simulink model "SingleTrack"  (Simulink 10.3)
settings: Solver=ode45  StartTime=0.0  StopTime=inf  FixedStep=0.001  RelTol=1e-3
PreLoadFcn:
  | SingleTrack_params
undefined symbols (not defined in the file): Car_Bdy1_mass, Car_Steering_i, Car_Whl_Radius, Car_WhlBaseF, Car_WhlBaseR, mEngineMax, PT_DL_iDiff, PT_GearBox_iForwardGears
libraries: CarMaker4SL x9
(part 3 of 4)

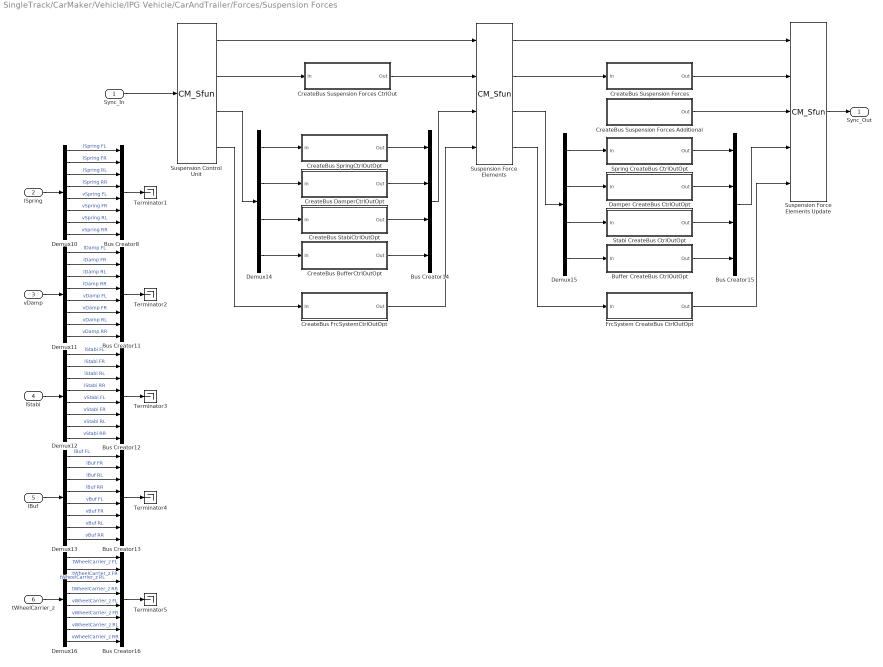
== system SingleTrack/CarMaker/Vehicle/IPG Vehicle/CarAndTrailer/Forces/Suspension Forces ==
  Sync_In : Inport
  lSpring : Inport  Port=2
  vDamp : Inport  Port=3
  lStabi : Inport  Port=4
  lBuf : Inport  Port=5
  tWheelCarrier_z : Inport  Port=6
  Buffer CreateBus CtrlOutOpt : Subsystem
  Bus Creator{8,11..13,16} (5 alike) : BusCreator  Inputs=8
  Bus Creator14 : BusCreator  Inputs=4
  Bus Creator15 : BusCreator  Inputs=4
  CreateBus BufferCtrlOutOpt : Subsystem
  CreateBus DamperCtrlOutOpt : Subsystem
  CreateBus FrcSystemCtrlOutOpt : Subsystem
  CreateBus SpringCtrlOutOpt : Subsystem
  CreateBus StabiCtrlOutOpt : Subsystem
  CreateBus Suspension Forces : Subsystem
  CreateBus Suspension Forces Additional : Subsystem
  CreateBus Suspension Forces CtrlOut : Subsystem
  Damper CreateBus CtrlOutOpt : Subsystem
  Demux{10..13,16} (5 alike) : Demux  Outputs=8
      settings: DisplayOption=none
  Demux14 : Demux
      settings: DisplayOption=none
  Demux15 : Demux
      settings: DisplayOption=none
  FrcSystem CreateBus CtrlOutOpt : Subsystem
  Spring CreateBus CtrlOutOpt : Subsystem
  Stabi CreateBus CtrlOutOpt : Subsystem
  Suspension Control Unit : S-Function  FunctionName=CM_Sfun  Parameters='ForcesSuspControl'  SFunctionDeploymentMode=off  EnableBusSupport=off
  Suspension Force Elements : S-Function  FunctionName=CM_Sfun  Parameters='ForcesSusp'  SFunctionDeploymentMode=off  EnableBusSupport=off
  Suspension Force Elements Update : S-Function  FunctionName=CM_Sfun  Parameters='ForcesSuspUpd'  SFunctionDeploymentMode=off  EnableBusSupport=off
  Terminator{1..5} (5 alike) : Terminator
  Sync_Out : Outport  VectorParamsAs1DForOutWhenUnconnected=off
  wires:
  Sync_In/1 -> Suspension Control Unit/1
  Suspension Control Unit/1 -> Suspension Force Elements/1
  Suspension Force Elements/1 -> Suspension Force Elements Update/1
  Suspension Force Elements Update/1 -> Sync_Out/1
  Demux13/4 -> Bus Creator13/4  "lBuf RR"
  Demux11/2 -> Bus Creator11/2  "lDamp FR"
  Demux13/8 -> Bus Creator13/8  "vBuf RR"
  Demux10/3 -> Bus Creator8/3  "lSpring RL"
  Demux10/1 -> Bus Creator8/1  "lSpring FL"
  vDamp/1 -> Demux11/1
  Demux13/2 -> Bus Creator13/2  "lBuf FR"
  Demux10/5 -> Bus Creator8/5  "vSpring FL"
  Bus Creator12/1 -> Terminator3/1
  Demux12/7 -> Bus Creator12/7  "vStabi RL"
  Demux10/4 -> Bus Creator8/4  "lSpring RR"
  Demux12/2 -> Bus Creator12/2  "lStabi FR"
  Demux11/5 -> Bus Creator11/5  "vDamp FL"
  Demux10/8 -> Bus Creator8/8  "vSpring RR"
  Demux12/1 -> Bus Creator12/1  "lStabi FL"
  Demux12/3 -> Bus Creator12/3  "lStabi RL"
  Demux11/6 -> Bus Creator11/6  "vDamp FR"
  lSpring/1 -> Demux10/1
  lBuf/1 -> Demux13/1
  Demux12/4 -> Bus Creator12/4  "lStabi RR"
  Bus Creator13/1 -> Terminator4/1
  Demux13/7 -> Bus Creator13/7  "vBuf RL"
  Demux12/8 -> Bus Creator12/8  "vStabi RR"
  Demux10/7 -> Bus Creator8/7  "vSpring RL"
  Demux11/8 -> Bus Creator11/8  "vDamp RR"
  Demux12/6 -> Bus Creator12/6  "vStabi FR"
  Demux11/1 -> Bus Creator11/1  "lDamp FL"
  Demux11/7 -> Bus Creator11/7  "vDamp RL"
  lStabi/1 -> Demux12/1
  Demux12/5 -> Bus Creator12/5  "vStabi FL"
  Bus Creator8/1 -> Terminator1/1
  Bus Creator11/1 -> Terminator2/1
  Demux13/1 -> Bus Creator13/1  "lBuf FL"
  Demux13/6 -> Bus Creator13/6  "vBuf FR"
  Demux11/4 -> Bus Creator11/4  "lDamp RR"
  Demux13/5 -> Bus Creator13/5  "vBuf FL"
  Demux10/6 -> Bus Creator8/6  "vSpring FR"
  Demux11/3 -> Bus Creator11/3  "lDamp RL"
  Demux10/2 -> Bus Creator8/2  "lSpring FR"
  Demux13/3 -> Bus Creator13/3  "lBuf RL"
  Suspension Force Elements/4 -> FrcSystem CreateBus CtrlOutOpt/1(In)
  FrcSystem CreateBus CtrlOutOpt/1(Out) -> Suspension Force Elements Update/5
  CreateBus SpringCtrlOutOpt/1(Out) -> Bus Creator14/1
  Demux14/1 -> CreateBus SpringCtrlOutOpt/1(In)
  Demux14/2 -> CreateBus DamperCtrlOutOpt/1(In)
  CreateBus DamperCtrlOutOpt/1(Out) -> Bus Creator14/2
  Demux14/3 -> CreateBus StabiCtrlOutOpt/1(In)
  CreateBus StabiCtrlOutOpt/1(Out) -> Bus Creator14/3
  CreateBus BufferCtrlOutOpt/1(Out) -> Bus Creator14/4
  Demux14/4 -> CreateBus BufferCtrlOutOpt/1(In)
  Demux15/4 -> Buffer CreateBus CtrlOutOpt/1(In)
  Buffer CreateBus CtrlOutOpt/1(Out) -> Bus Creator15/4
  Demux15/3 -> Stabi CreateBus CtrlOutOpt/1(In)
  Stabi CreateBus CtrlOutOpt/1(Out) -> Bus Creator15/3
  Demux15/2 -> Damper CreateBus CtrlOutOpt/1(In)
  Damper CreateBus CtrlOutOpt/1(Out) -> Bus Creator15/2
  Demux15/1 -> Spring CreateBus CtrlOutOpt/1(In)
  Spring CreateBus CtrlOutOpt/1(Out) -> Bus Creator15/1
  Suspension Force Elements/3 -> Demux15/1
  Bus Creator15/1 -> Suspension Force Elements Update/4
  Demux16/1 -> Bus Creator16/1  "tWheelCarrier_z FL"
  Demux16/6 -> Bus Creator16/6  "vWheelCarrier_z FR"
  Bus Creator16/1 -> Terminator5/1
  Demux16/2 -> Bus Creator16/2  "tWheelCarrier_z FR"
  Demux16/4 -> Bus Creator16/4  "tWheelCarrier_z RR"
  Demux16/8 -> Bus Creator16/8  "vWheelCarrier_z RR"
  Demux16/7 -> Bus Creator16/7  "vWheelCarrier_z RL"
  Demux16/3 -> Bus Creator16/3  "tWheelCarrier_z RL"
  Demux16/5 -> Bus Creator16/5  "vWheelCarrier_z FL"
  tWheelCarrier_z/1 -> Demux16/1
  CreateBus Suspension Forces Additional/1(Out) -> Suspension Force Elements Update/3
  Suspension Force Elements/2 -> CreateBus Suspension Forces/1(In)
  CreateBus Suspension Forces/1(Out) -> Suspension Force Elements Update/2
  Suspension Control Unit/2 -> CreateBus Suspension Forces CtrlOut/1(In)
  Suspension Control Unit/3 -> Demux14/1
  Suspension Control Unit/4 -> CreateBus FrcSystemCtrlOutOpt/1(In)
  CreateBus FrcSystemCtrlOutOpt/1(Out) -> Suspension Force Elements/4
  Bus Creator14/1 -> Suspension Force Elements/3
  CreateBus Suspension Forces CtrlOut/1(Out) -> Suspension Force Elements/2

== system SingleTrack/CarMaker/Vehicle/IPG Vehicle/CarAndTrailer/Forces/Tires ==
  note: The TireXX_Out signals will only be used if FileIdent is "CarMaker-Tire-CM4SL" in the tire parameter file!
      | An example parameter file can be found in Data/Tire/DT_CM4SL_UserTire.
  Sync_In : Inport
  TireFL_In : Inport  Port=2
  TireFR_In : Inport  Port=3
  TireRL_In : Inport  Port=4
  TireRR_In : Inport  Port=5
  Bus Creator{1..4} (4 alike) : BusCreator  Inputs=11
  Demux{1..3,8} (4 alike) : Demux  Outputs=7
      settings: DisplayOption=none
  TireFL : Subsystem
  TireFR : Subsystem
  TireRL : Subsystem
  TireRR : Subsystem
  TireFL_Out : Outport  VectorParamsAs1DForOutWhenUnconnected=off
  TireFR_Out : Outport  Port=2  VectorParamsAs1DForOutWhenUnconnected=off
  TireRL_Out : Outport  Port=3  VectorParamsAs1DForOutWhenUnconnected=off
  TireRR_Out : Outport  Port=4  VectorParamsAs1DForOutWhenUnconnected=off
  wires:
  Sync_In/1 -> TireRR/1(Sync_In), TireRL/1(Sync_In), TireFR/1(Sync_In), TireFL/1(Sync_In)
  Bus Creator4/1 -> TireRR_Out/1
  Bus Creator2/1 -> TireRL_Out/1
  Bus Creator1/1 -> TireFR_Out/1
  Demux3/5 -> TireRR/6(Rim_turnv)  "Tire_In Rim_turnv"
  Demux3/4 -> TireRR/5(Rim_rotv)  "Tire_In Rim_rotv"
  Demux3/1 -> TireRR/2(Load)  "Tire_In Load"
  Demux3/7 -> TireRR/8(muRoad)  "Tire_In mu"
  Demux3/6 -> TireRR/7(InclinAngle)  "Tire_In Camber"
  Demux3/2 -> TireRR/3(vxtrans)  "Tire_In vxtrans"
  Demux3/3 -> TireRR/4(vytrans)  "Tire_In vytrans"
  TireRR/11(AlignTrq) -> Bus Creator4/11  "Tire_Out AlignTrq"
  TireRR/10(RollResist) -> Bus Creator4/10  "Tire_Out RollResist"
  TireRR/9(OverturnTrq) -> Bus Creator4/9  "Tire_Out OverturnTrq"
  TireRR/8(LoadFrc) -> Bus Creator4/8  "Tire_Out LoadFrc"
  TireRR/7(SideFrc) -> Bus Creator4/7  "Tire_Out SideFrc"
  TireRR/6(LongFrc) -> Bus Creator4/6  "Tire_Out LongFrc"
  TireRR/5(vBelt) -> Bus Creator4/5  "Tire_Out vBelt"
  TireRR/4(rBelt_eff) -> Bus Creator4/4  "Tire_Out rBelt_eff"
  TireRR/3(TurnSlp) -> Bus Creator4/3  "Tire_Out TurnSlp"
  TireRR/1(Slp) -> Bus Creator4/1  "Tire_Out Slp"
  TireRR/2(Alpha) -> Bus Creator4/2  "Tire_Out Alpha"
  Demux2/5 -> TireRL/6(Rim_turnv)  "Tire_In Rim_turnv"
  Demux2/4 -> TireRL/5(Rim_rotv)  "Tire_In Rim_rotv"
  Demux2/1 -> TireRL/2(Load)  "Tire_In Load"
  Demux2/7 -> TireRL/8(muRoad)  "Tire_In mu"
  Demux2/6 -> TireRL/7(InclinAngle)  "Tire_In Camber"
  Demux2/2 -> TireRL/3(vxtrans)  "Tire_In vxtrans"
  Demux2/3 -> TireRL/4(vytrans)  "Tire_In vytrans"
  TireRL/11(AlignTrq) -> Bus Creator2/11  "Tire_Out AlignTrq"
  TireRL/10(RollResist) -> Bus Creator2/10  "Tire_Out RollResist"
  TireRL/9(OverturnTrq) -> Bus Creator2/9  "Tire_Out OverturnTrq"
  TireRL/8(LoadFrc) -> Bus Creator2/8  "Tire_Out LoadFrc"
  TireRL/7(SideFrc) -> Bus Creator2/7  "Tire_Out SideFrc"
  TireRL/6(LongFrc) -> Bus Creator2/6  "Tire_Out LongFrc"
  TireRL/5(vBelt) -> Bus Creator2/5  "Tire_Out vBelt"
  TireRL/4(rBelt_eff) -> Bus Creator2/4  "Tire_Out rBelt_eff"
  TireRL/3(TurnSlp) -> Bus Creator2/3  "Tire_Out TurnSlp"
  TireRL/1(Slp) -> Bus Creator2/1  "Tire_Out Slp"
  TireRL/2(Alpha) -> Bus Creator2/2  "Tire_Out Alpha"
  Demux1/5 -> TireFR/6(Rim_turnv)  "Tire_In Rim_turnv"
  Demux1/4 -> TireFR/5(Rim_rotv)  "Tire_In Rim_rotv"
  Demux1/1 -> TireFR/2(Load)  "Tire_In Load"
  Demux1/7 -> TireFR/8(muRoad)  "Tire_In mu"
  Demux1/6 -> TireFR/7(InclinAngle)  "Tire_In Camber"
  Demux1/2 -> TireFR/3(vxtrans)  "Tire_In vxtrans"
  Demux1/3 -> TireFR/4(vytrans)  "Tire_In vytrans"
  TireFR/11(AlignTrq) -> Bus Creator1/11  "Tire_Out AlignTrq"
  TireFR/10(RollResist) -> Bus Creator1/10  "Tire_Out RollResist"
  TireFR/9(OverturnTrq) -> Bus Creator1/9  "Tire_Out OverturnTrq"
  TireFR/8(LoadFrc) -> Bus Creator1/8  "Tire_Out LoadFrc"
  TireFR/7(SideFrc) -> Bus Creator1/7  "Tire_Out SideFrc"
  TireFR/6(LongFrc) -> Bus Creator1/6  "Tire_Out LongFrc"
  TireFR/5(vBelt) -> Bus Creator1/5  "Tire_Out vBelt"
  TireFR/4(rBelt_eff) -> Bus Creator1/4  "Tire_Out rBelt_eff"
  TireFR/3(TurnSlp) -> Bus Creator1/3  "Tire_Out TurnSlp"
  TireFR/1(Slp) -> Bus Creator1/1  "Tire_Out Slp"
  TireFR/2(Alpha) -> Bus Creator1/2  "Tire_Out Alpha"
  Demux8/5 -> TireFL/6(Rim_turnv)  "Tire_In Rim_turnv"
  Demux8/4 -> TireFL/5(Rim_rotv)  "Tire_In Rim_rotv"
  TireFL_In/1 -> Demux8/1
  Demux8/1 -> TireFL/2(Load)  "Tire_In Load"
  Demux8/7 -> TireFL/8(muRoad)  "Tire_In mu"
  Demux8/6 -> TireFL/7(InclinAngle)  "Tire_In Camber"
  Demux8/2 -> TireFL/3(vxtrans)  "Tire_In vxtrans"
  Demux8/3 -> TireFL/4(vytrans)  "Tire_In vytrans"
  TireFL/11(AlignTrq) -> Bus Creator3/11  "Tire_Out AlignTrq"
  TireFL/10(RollResist) -> Bus Creator3/10  "Tire_Out RollResist"
  TireFL/9(OverturnTrq) -> Bus Creator3/9  "Tire_Out OverturnTrq"
  TireFL/8(LoadFrc) -> Bus Creator3/8  "Tire_Out LoadFrc"
  TireFL/7(SideFrc) -> Bus Creator3/7  "Tire_Out SideFrc"
  TireFL/6(LongFrc) -> Bus Creator3/6  "Tire_Out LongFrc"
  TireFL/5(vBelt) -> Bus Creator3/5  "Tire_Out vBelt"
  TireFL/4(rBelt_eff) -> Bus Creator3/4  "Tire_Out rBelt_eff"
  TireFL/3(TurnSlp) -> Bus Creator3/3  "Tire_Out TurnSlp"
  TireFL/1(Slp) -> Bus Creator3/1  "Tire_Out Slp"
  TireFL/2(Alpha) -> Bus Creator3/2  "Tire_Out Alpha"
  Bus Creator3/1 -> TireFL_Out/1
  TireFR_In/1 -> Demux1/1
  TireRL_In/1 -> Demux2/1
  TireRR_In/1 -> Demux3/1

== system SingleTrack/CarMaker/Vehicle/IPG Vehicle/CarAndTrailer/Forces/Vehicle Forces ==
  Sync_In : Inport
  Bus Creator1 : BusCreator  Inputs=12
  Bus Creator8 : BusCreator  Inputs=16
  BusCreator1 : BusCreator  Inputs=4
  BusCreator2 : BusCreator  Inputs=9
  Demux : Demux  Outputs=16
      settings: DisplayOption=none
  Demux1 : Demux  Outputs=12
      settings: DisplayOption=none
  Demux2 : Demux  Outputs=13
      settings: DisplayOption=none
  Forces : S-Function  FunctionName=CM_Sfun  Parameters='Forces'  SFunctionDeploymentMode=off  EnableBusSupport=off
  Terminator : Terminator
  Sync_Out : Outport  VectorParamsAs1DForOutWhenUnconnected=off
  Car.Virtual : Outport  Port=2  VectorParamsAs1DForOutWhenUnconnected=off
  Car.Aero : Outport  Port=3  VectorParamsAs1DForOutWhenUnconnected=off
  Car.Load : Outport  Port=4  VectorParamsAs1DForOutWhenUnconnected=off
  wires:
  BusCreator1/1 -> Terminator/1  "Aero IF (in)"
  Demux2/13 -> BusCreator2/9  "car Aero Trq_1 z"
  Demux2/12 -> BusCreator2/8  "car Aero Trq_1 y"
  Demux2/11 -> BusCreator2/7  "car Aero Trq_1 x"
  Demux2/10 -> BusCreator2/6  "car Aero Frc_1 z"
  Demux2/9 -> BusCreator2/5  "car Aero Frc_1 y"
  Demux2/8 -> BusCreator2/4  "car Aero Frc_1 x"
  Demux2/7 -> BusCreator2/3  "car Aero PoA_1 z"
  Demux2/6 -> BusCreator2/2  "car Aero PoA_1 y"
  Demux2/5 -> BusCreator2/1  "car Aero PoA_1 x"
  Demux2/4 -> BusCreator1/4  "car Aero tau_1"
  Demux2/3 -> BusCreator1/3  "car Aero ApproachVel_1 z"
  Demux2/2 -> BusCreator1/2  "car Aero ApproachVel_1 y"
  Demux2/1 -> BusCreator1/1  "car Aero ApproachVel_1 x"
  Demux/16 -> Bus Creator8/16  "Car Load_3 tz"
  Demux/15 -> Bus Creator8/15  "Car Load_3 ty"
  Demux/14 -> Bus Creator8/14  "Car Load_3 tx"
  Demux/13 -> Bus Creator8/13  "Car Load_3 mass"
  Demux1/12 -> Bus Creator1/12  "Car Virtual Trq_0 z"
  Demux1/11 -> Bus Creator1/11  "Car Virtual Trq_0 y"
  Demux1/10 -> Bus Creator1/10  "Car Virtual Trq_0 x"
  Demux1/9 -> Bus Creator1/9  "Car Virtual Trq_1 z"
  Demux1/8 -> Bus Creator1/8  "Car Virtual Trq_1 y"
  Demux1/7 -> Bus Creator1/7  "Car Virtual Trq_1 x"
  Demux1/6 -> Bus Creator1/6  "Car Virtual Frc_0 z"
  Demux1/5 -> Bus Creator1/5  "Car Virtual Frc_0 y"
  Demux1/4 -> Bus Creator1/4  "Car Virtual Frc_0 x"
  Sync_In/1 -> Forces/1
  Forces/1 -> Sync_Out/1
  BusCreator2/1 -> Car.Aero/1
  Demux1/1 -> Bus Creator1/1  "Car Virtual Frc_1 x"
  Demux1/2 -> Bus Creator1/2  "Car Virtual Frc_1 y"
  Demux1/3 -> Bus Creator1/3  "Car Virtual Frc_1 z"
  Forces/3 -> Demux2/1
  Forces/2 -> Demux1/1
  Bus Creator1/1 -> Car.Virtual/1
  Bus Creator8/1 -> Car.Load/1
  Demux/1 -> Bus Creator8/1  "Car Load_0 mass"
  Demux/2 -> Bus Creator8/2  "Car Load_0 tx"
  Demux/3 -> Bus Creator8/3  "Car Load_0 ty"
  Demux/4 -> Bus Creator8/4  "Car Load_0 tz"
  Demux/5 -> Bus Creator8/5  "Car Load_1 mass"
  Demux/6 -> Bus Creator8/6  "Car Load_1 tx"
  Demux/7 -> Bus Creator8/7  "Car Load_1 ty"
  Demux/8 -> Bus Creator8/8  "Car Load_1 tz"
  Demux/9 -> Bus Creator8/9  "Car Load_2 mass"
  Demux/10 -> Bus Creator8/10  "Car Load_2 tx"
  Demux/11 -> Bus Creator8/11  "Car Load_2 ty"
  Demux/12 -> Bus Creator8/12  "Car Load_2 tz"
  Forces/4 -> Demux/1

== system SingleTrack/CarMaker/Vehicle/IPG Vehicle/CarAndTrailer/Trailer/CreateBus Car.Hitch.FrcTrq ==
  In1 : Inport
  Bus Creator7 : BusCreator  Inputs=6
  Demux7 : Demux  Outputs=6
      settings: DisplayOption=none
  Out1 : Outport  VectorParamsAs1DForOutWhenUnconnected=off
  wires:
  In1/1 -> Demux7/1
  Bus Creator7/1 -> Out1/1
  Demux7/6 -> Bus Creator7/6  "Car Hitch Trq2Car z"
  Demux7/5 -> Bus Creator7/5  "Car Hitch Trq2Car y"
  Demux7/4 -> Bus Creator7/4  "Car Hitch Trq2Car x"
  Demux7/3 -> Bus Creator7/3  "Car Hitch Frc2Car z"
  Demux7/2 -> Bus Creator7/2  "Car Hitch Frc2Car y"
  Demux7/1 -> Bus Creator7/1  "Car Hitch Frc2Car x"

== system SingleTrack/CarMaker/Vehicle/IPG Vehicle/CarAndTrailer/Trailer/CreateBus Vhcl.Motion ==
  In1 : Inport
  BusCreator : BusCreator  Inputs=15
  Demux : Demux  Outputs=15
      settings: DisplayOption=none
  Out1 : Outport  VectorParamsAs1DForOutWhenUnconnected=off
  wires:
  Demux/15 -> BusCreator/15  "Vhcl YawAcc"
  Demux/14 -> BusCreator/14  "Vhcl YawVel"
  Demux/13 -> BusCreator/13  "Vhcl Yaw"
  Demux/12 -> BusCreator/12  "Vhcl PitchAcc"
  Demux/11 -> BusCreator/11  "Vhcl PitchVel"
  Demux/10 -> BusCreator/10  "Vhcl Pitch"
  Demux/9 -> BusCreator/9  "Vhcl RollAcc"
  Demux/8 -> BusCreator/8  "Vhcl RollVel"
  Demux/7 -> BusCreator/7  "Vhcl Roll"
  Demux/6 -> BusCreator/6  "Vhcl Hitch_Pos z"
  Demux/5 -> BusCreator/5  "Vhcl Hitch_Pos y"
  Demux/4 -> BusCreator/4  "Vhcl Hitch_Pos x"
  Demux/3 -> BusCreator/3  "Vhcl sRoad"
  Demux/2 -> BusCreator/2  "Vhcl Distance"
  Demux/1 -> BusCreator/1  "Vhcl v"
  In1/1 -> Demux/1
  BusCreator/1 -> Out1/1

== system SingleTrack/CarMaker/Vehicle/IPG Vehicle/CarAndTrailer/Trailer/CreateBus Vhcl.PoI ==
  In1 : Inport
  Bus Creator3 : BusCreator  Inputs=18
  Demux3 : Demux  Outputs=18
      settings: DisplayOption=none
  Out1 : Outport  VectorParamsAs1DForOutWhenUnconnected=off
  wires:
  Demux3/18 -> Bus Creator3/18  "Vhcl PoI_GCS Elev"
  Demux3/17 -> Bus Creator3/17  "Vhcl PoI_GCS Lat"
  Demux3/16 -> Bus Creator3/16  "Vhcl PoI_GCS Long"
  Demux3/15 -> Bus Creator3/15  "Vhcl PoI_Acc_1 z"
  Demux3/14 -> Bus Creator3/14  "Vhcl PoI_Acc_1 y"
  Demux3/13 -> Bus Creator3/13  "Vhcl PoI_Acc_1 x"
  Demux3/12 -> Bus Creator3/12  "Vhcl PoI_Vel_1 z"
  Demux3/11 -> Bus Creator3/11  "Vhcl PoI_Vel_1 y"
  Demux3/10 -> Bus Creator3/10  "Vhcl PoI_Vel_1 x"
  Demux3/9 -> Bus Creator3/9  "Vhcl PoI_Acc z"
  Demux3/8 -> Bus Creator3/8  "Vhcl PoI_Acc y"
  Demux3/7 -> Bus Creator3/7  "Vhcl PoI_Acc x"
  Demux3/6 -> Bus Creator3/6  "Vhcl PoI_Vel z"
  Demux3/5 -> Bus Creator3/5  "Vhcl PoI_Vel y"
  Demux3/4 -> Bus Creator3/4  "Vhcl PoI_Vel x"
  Demux3/3 -> Bus Creator3/3  "Vhcl PoI_Pos z"
  Demux3/2 -> Bus Creator3/2  "Vhcl PoI_Pos y"
  In1/1 -> Demux3/1
  Bus Creator3/1 -> Out1/1
  Demux3/1 -> Bus Creator3/1  "Vhcl PoI_Pos x"

== system SingleTrack/CarMaker/Vehicle/IPG Vehicle/CarAndTrailer/Trailer/CreateBus Vhcl.Steering ==
  In1 : Inport
  Bus Creator3 : BusCreator  Inputs=4
  Demux : Demux
      settings: DisplayOption=none
  Out1 : Outport  VectorParamsAs1DForOutWhenUnconnected=off
  wires:
  Bus Creator3/1 -> Out1/1
  Demux/1 -> Bus Creator3/1  "Vhcl Steering Ang"
  Demux/3 -> Bus Creator3/3  "Vhcl Steering AngAcc"
  Demux/2 -> Bus Creator3/2  "Vhcl Steering AngVel"
  Demux/4 -> Bus Creator3/4  "Vhcl Steering Trq"
  In1/1 -> Demux/1

== system SingleTrack/CarMaker/Vehicle/IPG Vehicle/CarAndTrailer/Trailer/CreateBus Vhcl.Wheel.FL ==
  In1 : Inport
  Bus Creator3 : BusCreator  Inputs=14
  Demux3 : Demux  Outputs=14
      settings: DisplayOption=none
  Out1 : Outport  VectorParamsAs1DForOutWhenUnconnected=off
  wires:
  Demux3/14 -> Bus Creator3/14  "Vhcl Wheel FL Trq_WhlBearing"
  Demux3/13 -> Bus Creator3/13  "Vhcl Wheel FL Trq_T2W"
  Demux3/12 -> Bus Creator3/12  "Vhcl Wheel FL SideSlip"
  Demux3/11 -> Bus Creator3/11  "Vhcl Wheel FL LongSlip"
  Demux3/10 -> Bus Creator3/10  "Vhcl Wheel FL vBelt"
  Demux3/9 -> Bus Creator3/9  "Vhcl Wheel FL Fz"
  Demux3/8 -> Bus Creator3/8  "Vhcl Wheel FL Fy"
  Demux3/7 -> Bus Creator3/7  "Vhcl Wheel FL Fx"
  Demux3/6 -> Bus Creator3/6  "Vhcl Wheel FL r_zxy z"
  Demux3/5 -> Bus Creator3/5  "Vhcl Wheel FL r_zxy y"
  Demux3/4 -> Bus Creator3/4  "Vhcl Wheel FL r_zxy x"
  Demux3/3 -> Bus Creator3/3  "Vhcl Wheel FL t z"
  Demux3/2 -> Bus Creator3/2  "Vhcl Wheel FL t y"
  In1/1 -> Demux3/1
  Bus Creator3/1 -> Out1/1
  Demux3/1 -> Bus Creator3/1  "Vhcl Wheel FL t x"

== system SingleTrack/CarMaker/Vehicle/IPG Vehicle/CarAndTrailer/Trailer/CreateBus Vhcl.Wheel.FR ==
  In1 : Inport
  Bus Creator3 : BusCreator  Inputs=14
  Demux3 : Demux  Outputs=14
      settings: DisplayOption=none
  Out1 : Outport  VectorParamsAs1DForOutWhenUnconnected=off
  wires:
  Demux3/14 -> Bus Creator3/14  "Vhcl Wheel FR Trq_WhlBearing"
  Demux3/13 -> Bus Creator3/13  "Vhcl Wheel FR Trq_T2W"
  Demux3/12 -> Bus Creator3/12  "Vhcl Wheel FR SideSlip"
  Demux3/11 -> Bus Creator3/11  "Vhcl Wheel FR LongSlip"
  Demux3/10 -> Bus Creator3/10  "Vhcl Wheel FR vBelt"
  Demux3/9 -> Bus Creator3/9  "Vhcl Wheel FR Fz"
  Demux3/8 -> Bus Creator3/8  "Vhcl Wheel FR Fy"
  Demux3/7 -> Bus Creator3/7  "Vhcl Wheel FR Fx"
  Demux3/6 -> Bus Creator3/6  "Vhcl Wheel FR r_zxy z"
  Demux3/5 -> Bus Creator3/5  "Vhcl Wheel FR r_zxy y"
  Demux3/4 -> Bus Creator3/4  "Vhcl Wheel FR r_zxy x"
  Demux3/3 -> Bus Creator3/3  "Vhcl Wheel FR t z"
  Demux3/2 -> Bus Creator3/2  "Vhcl Wheel FR t y"
  In1/1 -> Demux3/1
  Bus Creator3/1 -> Out1/1
  Demux3/1 -> Bus Creator3/1  "Vhcl Wheel FR t x"

== system SingleTrack/CarMaker/Vehicle/IPG Vehicle/CarAndTrailer/Trailer/CreateBus Vhcl.Wheel.RL ==
  In1 : Inport
  Bus Creator3 : BusCreator  Inputs=14
  Demux3 : Demux  Outputs=14
      settings: DisplayOption=none
  Out1 : Outport  VectorParamsAs1DForOutWhenUnconnected=off
  wires:
  Demux3/14 -> Bus Creator3/14  "Vhcl Wheel RL Trq_WhlBearing"
  Demux3/13 -> Bus Creator3/13  "Vhcl Wheel RL Trq_T2W"
  Demux3/12 -> Bus Creator3/12  "Vhcl Wheel RL SideSlip"
  Demux3/11 -> Bus Creator3/11  "Vhcl Wheel RL LongSlip"
  Demux3/10 -> Bus Creator3/10  "Vhcl Wheel RL vBelt"
  Demux3/9 -> Bus Creator3/9  "Vhcl Wheel RL Fz"
  Demux3/8 -> Bus Creator3/8  "Vhcl Wheel RL Fy"
  Demux3/7 -> Bus Creator3/7  "Vhcl Wheel RL Fx"
  Demux3/6 -> Bus Creator3/6  "Vhcl Wheel RL r_zxy z"
  Demux3/5 -> Bus Creator3/5  "Vhcl Wheel RL r_zxy y"
  Demux3/4 -> Bus Creator3/4  "Vhcl Wheel RL r_zxy x"
  Demux3/3 -> Bus Creator3/3  "Vhcl Wheel RL t z"
  Demux3/2 -> Bus Creator3/2  "Vhcl Wheel RL t y"
  In1/1 -> Demux3/1
  Bus Creator3/1 -> Out1/1
  Demux3/1 -> Bus Creator3/1  "Vhcl Wheel RL t x"

== system SingleTrack/CarMaker/Vehicle/IPG Vehicle/CarAndTrailer/Trailer/CreateBus Vhcl.Wheel.RR ==
  In1 : Inport
  Bus Creator3 : BusCreator  Inputs=14
  Demux3 : Demux  Outputs=14
      settings: DisplayOption=none
  Out1 : Outport  VectorParamsAs1DForOutWhenUnconnected=off
  wires:
  Demux3/14 -> Bus Creator3/14  "Vhcl Wheel RR Trq_WhlBearing"
  Demux3/13 -> Bus Creator3/13  "Vhcl Wheel RR Trq_T2W"
  Demux3/12 -> Bus Creator3/12  "Vhcl Wheel RR SideSlip"
  Demux3/11 -> Bus Creator3/11  "Vhcl Wheel RR LongSlip"
  Demux3/10 -> Bus Creator3/10  "Vhcl Wheel RR vBelt"
  Demux3/9 -> Bus Creator3/9  "Vhcl Wheel RR Fz"
  Demux3/8 -> Bus Creator3/8  "Vhcl Wheel RR Fy"
  Demux3/7 -> Bus Creator3/7  "Vhcl Wheel RR Fx"
  Demux3/6 -> Bus Creator3/6  "Vhcl Wheel RR r_zxy z"
  Demux3/5 -> Bus Creator3/5  "Vhcl Wheel RR r_zxy y"
  Demux3/4 -> Bus Creator3/4  "Vhcl Wheel RR r_zxy x"
  Demux3/3 -> Bus Creator3/3  "Vhcl Wheel RR t z"
  Demux3/2 -> Bus Creator3/2  "Vhcl Wheel RR t y"
  In1/1 -> Demux3/1
  Bus Creator3/1 -> Out1/1
  Demux3/1 -> Bus Creator3/1  "Vhcl Wheel RR t x"

== system SingleTrack/CarMaker/Vehicle/User Vehicle (CM4SL)/CarAndTrailer/CarAndTrailerUpd/CreateBus Brake.IF.In ==
  In : Inport
  BusCreator : BusCreator  Inputs=9
  Demux : Demux  Outputs=9
      settings: DisplayOption=none
  Out : Outport  VectorParamsAs1DForOutWhenUnconnected=off
  wires:
  Demux/9 -> BusCreator/9  "Brake IF Trq_Reg RR"
  Demux/8 -> BusCreator/8  "Brake IF Trq_Reg RL"
  Demux/7 -> BusCreator/7  "Brake IF Trq_Reg FR"
  Demux/6 -> BusCreator/6  "Brake IF Trq_Reg FL"
  Demux/5 -> BusCreator/5  "Brake IF Trq_Reg_max RR"
  Demux/4 -> BusCreator/4  "Brake IF Trq_Reg_max RL"
  Demux/3 -> BusCreator/3  "Brake IF Trq_Reg_max FR"
  Demux/2 -> BusCreator/2  "Brake IF Trq_Reg_max FL"
  Demux/1 -> BusCreator/1  "Brake IF T_env"
  BusCreator/1 -> Out/1
  In/1 -> Demux/1

== system SingleTrack/CarMaker/Vehicle/User Vehicle (CM4SL)/CarAndTrailer/CreateBus Vhcl.Fr1/BdyFrame2Vhcl.Fr1A ==
  note: Translate pseudo BdyFrame interface to Vhcl.Fr1
  t_0 : Inport
  v_0 : Inport  Port=2
  a_0 : Inport  Port=3
  omega_0 : Inport  Port=4
  alpha_0 : Inport  Port=5
  Tr2Fr0 : Inport  Port=6
  Bus Creator : BusCreator  Inputs=24
  Demux{,1..3,5} (5 alike) : Demux  Outputs=3
  Demux4 : Demux  Outputs=9
  Vhcl.Fr1 : Outport  VectorParamsAs1DForOutWhenUnconnected=off
  wires:
  t_0/1 -> Demux/1
  v_0/1 -> Demux1/1
  a_0/1 -> Demux2/1
  omega_0/1 -> Demux3/1
  alpha_0/1 -> Demux5/1
  Tr2Fr0/1 -> Demux4/1
  Demux4/9 -> Bus Creator/24  "Vhcl Fr1A_Tr2Fr0 22"
  Demux4/8 -> Bus Creator/23  "Vhcl Fr1A_Tr2Fr0 21"
  Demux4/7 -> Bus Creator/22  "Vhcl Fr1A_Tr2Fr0 20"
  Demux4/6 -> Bus Creator/21  "Vhcl Fr1A_Tr2Fr0 12"
  Demux4/5 -> Bus Creator/20  "Vhcl Fr1A_Tr2Fr0 11"
  Demux4/4 -> Bus Creator/19  "Vhcl Fr1A_Tr2Fr0 10"
  Demux4/3 -> Bus Creator/18  "Vhcl Fr1A_Tr2Fr0 02"
  Demux4/2 -> Bus Creator/17  "Vhcl Fr1A_Tr2Fr0 01"
  Demux4/1 -> Bus Creator/16  "Vhcl Fr1A_Tr2Fr0 00"
  Demux5/3 -> Bus Creator/15  "Vhcl Fr1A_alpha_0 z"
  Demux5/2 -> Bus Creator/14  "Vhcl Fr1A_alpha_0 y"
  Demux5/1 -> Bus Creator/13  "Vhcl Fr1A_alpha_0 x"
  Demux3/3 -> Bus Creator/12  "Vhcl Fr1A_omega_0 z"
  Demux3/2 -> Bus Creator/11  "Vhcl Fr1A_omega_0 y"
  Demux3/1 -> Bus Creator/10  "Vhcl Fr1A_omega_0 x"
  Demux2/3 -> Bus Creator/9  "Vhcl Fr1A_a_0 z"
  Demux2/2 -> Bus Creator/8  "Vhcl Fr1A_a_0 y"
  Demux2/1 -> Bus Creator/7  "Vhcl Fr1A_a_0 x"
  Demux1/3 -> Bus Creator/6  "Vhcl Fr1A_v_0 z"
  Demux1/2 -> Bus Creator/5  "Vhcl Fr1A_v_0 y"
  Demux1/1 -> Bus Creator/4  "Vhcl Fr1A_v_0 x"
  Demux/3 -> Bus Creator/3  "Vhcl Fr1A_t_0 z"
  Demux/2 -> Bus Creator/2  "Vhcl Fr1A_t_0 y"
  Demux/1 -> Bus Creator/1  "Vhcl Fr1 A_t_0 x"
  Bus Creator/1 -> Vhcl.Fr1/1

== system SingleTrack/CarMaker/Vehicle/User Vehicle (CM4SL)/CarAndTrailer/CreateBus Vhcl.Fr1/Tr2Fr0 ==
  Car : Inport
  Bus Creator : BusCreator  Inputs=9
  Subsystem_00 : Subsystem
  Subsystem_01 : Subsystem
  Subsystem_02 : Subsystem
  Subsystem_10 : Subsystem
  Subsystem_11 : Subsystem
  Subsystem_12 : Subsystem
  Subsystem_20 : Subsystem
  Subsystem_21 : Subsystem
  Subsystem_22 : Subsystem
  sincos : Subsystem
  Tr2Fr0 : Outport  VectorParamsAs1DForOutWhenUnconnected=off
  wires:
  Car/1 -> sincos/1(Car)
  sincos/1(sincos) -> Subsystem_10/1(sincos), Subsystem_11/1(sincos), Subsystem_20/1(sincos), Subsystem_21/1(sincos), Subsystem_22/1(sincos), Subsystem_12/1(sincos), Subsystem_00/1(sincos), Subsystem_01/1(sincos), Subsystem_02/1(sincos)
  Bus Creator/1 -> Tr2Fr0/1
  Subsystem_00/1(Tr2Fr1_00) -> Bus Creator/1  "Tr2Fr0_00"
  Subsystem_10/1(Tr2Fr1_10) -> Bus Creator/4  "Tr2Fr0_10"
  Subsystem_20/1(Tr2Fr1_20) -> Bus Creator/7  "Tr2Fr0_20"
  Subsystem_21/1(Tr2Fr1_21) -> Bus Creator/8  "Tr2Fr0_21"
  Subsystem_22/1(Tr2Fr1_22) -> Bus Creator/9  "Tr2Fr0_22"
  Subsystem_01/1(Tr2Fr1_01) -> Bus Creator/2  "Tr2Fr0_01"
  Subsystem_02/1(Tr2Fr1_02) -> Bus Creator/3  "Tr2Fr0_02"
  Subsystem_11/1(Tr2Fr1_11) -> Bus Creator/5  "Tr2Fr1_11"
  Subsystem_12/1(Tr2Fr1_12) -> Bus Creator/6  "Tr2Fr1_12"

== system SingleTrack/CarMaker/Vehicle/User Vehicle (CM4SL)/CarAndTrailer/CreateBus Vhcl.Fr1/a_0 ==
  Car : Inport
  Tr2Fr0 : Inport  Port=2
  Add : Sum
  Add1 : Sum
  Add2 : Sum
  Bus Selector1 : BusSelector  OutputSignals=Car_ax_1,Car_ay_1
  Bus Selector2 : BusSelector  OutputSignals=Tr2Fr0_00,Tr2Fr0_01,Tr2Fr0_10,Tr2Fr1_11,Tr2Fr0_20,Tr2Fr0_21
  Mux1 : Mux  Inputs=3
  Product{,1..5} (6 alike) : Product  RndMeth=Zero
  a_0 : Outport  VectorParamsAs1DForOutWhenUnconnected=off
  wires:
  Mux1/1 -> a_0/1
  Car/1 -> Bus Selector1/1
  Tr2Fr0/1 -> Bus Selector2/1
  Bus Selector1/2 -> Product/1, Product2/1, Product4/1  "<Car_ay_1>"
  Bus Selector1/1 -> Product1/1, Product3/1, Product5/1  "<Car_ax_1>"
  Product1/1 -> Add/1
  Product/1 -> Add/2
  Add/1 -> Mux1/1
  Product3/1 -> Add1/1
  Product2/1 -> Add1/2
  Bus Selector2/1 -> Product1/2  "<Tr2Fr0_00>"
  Bus Selector2/2 -> Product/2  "<Tr2Fr0_01>"
  Add1/1 -> Mux1/2
  Bus Selector2/3 -> Product3/2  "<Tr2Fr0_10>"
  Bus Selector2/4 -> Product2/2  "<Tr2Fr1_11>"
  Product5/1 -> Add2/1
  Product4/1 -> Add2/2
  Add2/1 -> Mux1/3
  Bus Selector2/6 -> Product4/2  "<Tr2Fr0_21>"
  Bus Selector2/5 -> Product5/2  "<Tr2Fr0_20>"

== system SingleTrack/CarMaker/Vehicle/User Vehicle (CM4SL)/CarAndTrailer/CreateBus Vhcl.Fr1/t_0 ==
  Car : Inport
  Bus Selector : BusSelector  OutputSignals=Car_x,Car_y,Road_Fr1_z
  Mux : Mux  Inputs=3
  t_0 : Outport  VectorParamsAs1DForOutWhenUnconnected=off
  wires:
  Bus Selector/1 -> Mux/1  "<Car_x>"
  Bus Selector/2 -> Mux/2  "<Car_y>"
  Bus Selector/3 -> Mux/3  "<Road_Fr1_z>"
  Car/1 -> Bus Selector/1
  Mux/1 -> t_0/1

== system SingleTrack/CarMaker/Vehicle/User Vehicle (CM4SL)/CarAndTrailer/CreateBus Vhcl.Fr1/v_0 ==
  Car : Inport
  Tr2Fr0 : Inport  Port=2
  Bus Selector1 : BusSelector  OutputSignals=Car_vx_1
  Bus Selector2 : BusSelector  OutputSignals=Tr2Fr0_00,Tr2Fr0_10,Tr2Fr0_20
  Mux1 : Mux  Inputs=3
  Product : Product  RndMeth=Zero
  Product1 : Product  RndMeth=Zero
  Product2 : Product  RndMeth=Zero
  v_0 : Outport  VectorParamsAs1DForOutWhenUnconnected=off
  wires:
  Car/1 -> Bus Selector1/1
  Mux1/1 -> v_0/1
  Tr2Fr0/1 -> Bus Selector2/1
  Bus Selector2/1 -> Product/2  "<Tr2Fr0_00>"
  Bus Selector2/2 -> Product1/2  "<Tr2Fr0_10>"
  Bus Selector2/3 -> Product2/2  "<Tr2Fr0_20>"
  Bus Selector1/1 -> Product/1, Product1/1, Product2/1  "<Car_vx_1>"
  Product/1 -> Mux1/1
  Product1/1 -> Mux1/2
  Product2/1 -> Mux1/3

== system SingleTrack/CarMaker/Vehicle/User Vehicle (CM4SL)/CarAndTrailer/PowerTrainUpd/Set OperationState ==
  note: Handles OperationState in Post-processing (SimCore.State >=9)
  If : If  IfExpression=u1 >= 9
  If Action Subsystem : Subsystem  TreatAsAtomicUnit=on
  If Action Subsystem1 : Subsystem  TreatAsAtomicUnit=on
  Merge : Merge
  Read CM Dict : CarMaker4SL/Read CM Dict  xname=SC.State  xsync=off  xstime=Continuous
  Read CM Dict1 : CarMaker4SL/Read CM Dict  xname=DM.OperationState_trg  xsync=off  xstime=Continuous
  OperationState : Outport  VectorParamsAs1DForOutWhenUnconnected=off
  wires:
  Merge/1 -> OperationState/1
  If/1 -> If Action Subsystem/Action
  If/2 -> If Action Subsystem1/Action
  If Action Subsystem/1(Out1) -> Merge/1
  If Action Subsystem1/1(Out1) -> Merge/2
  Read CM Dict/1 -> If/1
  Read CM Dict1/1 -> If Action Subsystem1/1(In1), If Action Subsystem/1(In1)

== system SingleTrack/CarMaker/Vehicle/User Vehicle (CM4SL)/CarAndTrailer/Query Road/IPGRoad5 ==
  rIn.st : Inport
  rIn.xyz : Inport  Port=2
  Bus Creator1 : BusCreator  Inputs=9
  Bus Creator2 : BusCreator  Inputs=22
  Demux1 : Demux  Outputs=9
  Demux3 : Demux  Outputs=22
  S-Function : S-Function  FunctionName=cm_road  Parameters=xname,xevalmode,xconsiderbumps,xusepath,xwithcurve,xabort  SFunctionDeploymentMode=off  EnableBusSupport=off
  rOutGeo : Outport  VectorParamsAs1DForOutWhenUnconnected=off
  rOutRoute : Outport  Port=2  VectorParamsAs1DForOutWhenUnconnected=off
  wires:
  Demux3/22 -> Bus Creator2/22  "fric"
  S-Function/2 -> Demux3/1
  S-Function/1 -> Demux1/1
  Bus Creator1/1 -> rOutGeo/1
  Demux1/9 -> Bus Creator1/9  "fric"
  Demux1/8 -> Bus Creator1/8  "onJunction"
  Demux1/7 -> Bus Creator1/7  "onRoad"
  Demux1/6 -> Bus Creator1/6  "nuv z"
  Demux1/5 -> Bus Creator1/5  "nuv y"
  Demux1/4 -> Bus Creator1/4  "nuv x"
  Demux1/3 -> Bus Creator1/3  "z"
  Demux1/2 -> Bus Creator1/2  "y"
  Demux1/1 -> Bus Creator1/1  "x"
  Demux3/21 -> Bus Creator2/21  "curveZ"
  Demux3/20 -> Bus Creator2/20  "slope"
  Demux3/19 -> Bus Creator2/19  "grade"
  Demux3/18 -> Bus Creator2/18  "onRoad"
  Demux3/17 -> Bus Creator2/17  "width right"
  Demux3/16 -> Bus Creator2/16  "width left"
  Demux3/15 -> Bus Creator2/15  "curveXY"
  Demux3/13 -> Bus Creator2/13  "s"
  Demux3/14 -> Bus Creator2/14  "t"
  Demux3/12 -> Bus Creator2/12  "tuv z"
  Demux3/11 -> Bus Creator2/11  "tuv y"
  Demux3/10 -> Bus Creator2/10  "tuv x"
  Demux3/9 -> Bus Creator2/9  "suv z"
  Demux3/8 -> Bus Creator2/8  "suv y"
  Demux3/7 -> Bus Creator2/7  "suv x"
  Demux3/6 -> Bus Creator2/6  "nuv z"
  Demux3/5 -> Bus Creator2/5  "nuv y"
  Demux3/4 -> Bus Creator2/4  "nuv x"
  Demux3/3 -> Bus Creator2/3  "z"
  Demux3/2 -> Bus Creator2/2  "y"
  Demux3/1 -> Bus Creator2/1  "x"
  Bus Creator2/1 -> rOutRoute/1
  rIn.xyz/1 -> S-Function/2
  rIn.st/1 -> S-Function/1

== system SingleTrack/CarMaker/Vehicle/User Vehicle (CM4SL)/CarAndTrailer/single-track mass point model/Car.v_1 ==
  ax : Inport
  Constant1 : Constant  Value=0.1
  PassIfSim : Subsystem
  Read CM Parameter : CarMaker4SL/Read CM Parameter  xfile=TestRun  xkey=DrivMan.Man.Start.Velocity  xnout=1  xdefaults=0  xmuxed=on  xstime=Continuous
  kmh2ms : Gain  Gain=1000/3600  OutDataTypeStr=Inherit: Inherit via back propagation  SaturateOnIntegerOverflow=on  ParamDataTypeStr=Inherit: Same as input
  vMin : MinMax  Function=max  Inputs=2  InputSameDT=on  SaturateOnIntegerOverflow=on
  v_dot * dt : Integrator  ExternalReset=level  InitialConditionSource=external  InitialCondition=22.222
  v_1 : Outport  VectorParamsAs1DForOutWhenUnconnected=off
  wires:
  Read CM Parameter/1 -> kmh2ms/1
  kmh2ms/1 -> vMin/2
  Constant1/1 -> vMin/1
  [TRStart] -> v_dot * dt/2
  vMin/1 -> v_dot * dt/3
  v_dot * dt/1 -> v_1/1
  ax/1 -> PassIfSim/1(In1)
  PassIfSim/1(Out1) -> v_dot * dt/1

== system SingleTrack/CarMaker/Vehicle/User Vehicle (CM4SL)/CarAndTrailer/single-track mass point model/PassIfSim ==
  note: Output original value only when simulating,
      | and zero during pre- or postprocessing.
  In1 : Inport
  "   " : Product  InputSameDT=on  SaturateOnIntegerOverflow=on  OutDataTypeStr=Inherit: Same as first input
  Data Type Conversion : DataTypeConversion
  Out1 : Outport  VectorParamsAs1DForOutWhenUnconnected=off
  wires:
  [TRSim] -> Data Type Conversion/1
  "   "/1 -> Out1/1
  Data Type Conversion/1 -> "   "/2
  In1/1 -> "   "/1

== system SingleTrack/CarMaker/Vehicle/User Vehicle (CM4SL)/CarAndTrailer/single-track mass point model/PassIfSim1 ==
  note: Output original value only when simulating,
      | and zero during pre- or postprocessing.
  In1 : Inport
  "   " : Product  InputSameDT=on  SaturateOnIntegerOverflow=on  OutDataTypeStr=Inherit: Same as first input
  Data Type Conversion : DataTypeConversion
  Out1 : Outport  VectorParamsAs1DForOutWhenUnconnected=off
  wires:
  [TRSim] -> Data Type Conversion/1
  "   "/1 -> Out1/1
  Data Type Conversion/1 -> "   "/2
  In1/1 -> "   "/1

== system SingleTrack/CarMaker/Vehicle/User Vehicle (CM4SL)/CarAndTrailer/single-track mass point model/PassIfSim2 ==
  note: Output original value only when simulating,
      | and zero during pre- or postprocessing.
  In1 : Inport
  "   " : Product  InputSameDT=on  SaturateOnIntegerOverflow=on  OutDataTypeStr=Inherit: Same as first input
  Data Type Conversion : DataTypeConversion
  Out1 : Outport  VectorParamsAs1DForOutWhenUnconnected=off
  wires:
  [TRSim] -> Data Type Conversion/1
  "   "/1 -> Out1/1
  Data Type Conversion/1 -> "   "/2
  In1/1 -> "   "/1

== system SingleTrack/CarMaker/Vehicle/User Vehicle (CM4SL)/CarAndTrailer/single-track mass point model/Vehicle Initial Cfg ==
  CreateBus Vhcl.Cfg : Subsystem
  VehicleControlUpd : S-Function  FunctionName=cm_initial  SFunctionDeploymentMode=off  EnableBusSupport=off
  Vhcl.Cfg : Outport  VectorParamsAs1DForOutWhenUnconnected=off
  wires:
  VehicleControlUpd/1 -> CreateBus Vhcl.Cfg/1(In1)
  CreateBus Vhcl.Cfg/1(Out1) -> Vhcl.Cfg/1

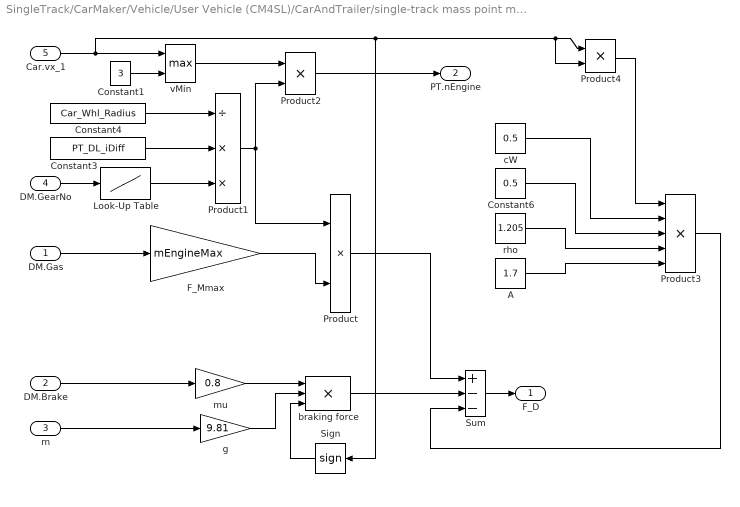
== system SingleTrack/CarMaker/Vehicle/User Vehicle (CM4SL)/CarAndTrailer/single-track mass point model/driving force ==
  DM.Gas : Inport
  DM.Brake : Inport  Port=2
  m : Inport  Port=3
  DM.GearNo : Inport  Port=4
  Car.vx_1 : Inport  Port=5
  A : Constant  Value=1.7
  Constant1 : Constant  Value=3
  Constant3 : Constant  Value=PT_DL_iDiff
  Constant4 : Constant  Value=Car_Whl_Radius
  Constant6 : Constant  Value=0.5
  "F_Mmax " : Gain  Gain=mEngineMax  SaturateOnIntegerOverflow=on  OutDataTypeStr=Inherit: Same as input  ParamDataTypeStr=Inherit: Same as input
  Look-Up Table : Lookup  InputValues=[0 1 2 3 4 5 6]  Table=PT_GearBox_iForwardGears  LookUpMeth=Interpolation-Use End Values  SaturateOnIntegerOverflow=on
  Product : Product  Inputs=**  InputSameDT=on  SaturateOnIntegerOverflow=on  OutDataTypeStr=Inherit: Same as first input
  Product1 : Product  Inputs=/**  InputSameDT=on  SaturateOnIntegerOverflow=on  OutDataTypeStr=Inherit: Same as first input
  Product2 : Product  InputSameDT=on  SaturateOnIntegerOverflow=on  OutDataTypeStr=Inherit: Same as first input
  Product3 : Product  Inputs=5  InputSameDT=on  SaturateOnIntegerOverflow=on  OutDataTypeStr=Inherit: Same as first input
  Product4 : Product  InputSameDT=on  SaturateOnIntegerOverflow=on  OutDataTypeStr=Inherit: Same as first input
  Sign : Signum  ZeroCross=off
  Sum : Sum  Inputs=+--  InputSameDT=on  SaturateOnIntegerOverflow=on  OutDataTypeStr=Inherit: Same as first input
  braking force : Product  Inputs=3  InputSameDT=on  SaturateOnIntegerOverflow=on  OutDataTypeStr=Inherit: Same as first input
  cW : Constant  Value=0.5
  g : Gain  Gain=9.81  SaturateOnIntegerOverflow=on  OutDataTypeStr=Inherit: Same as input  ParamDataTypeStr=Inherit: Same as input
  mu : Gain  Gain=0.8  SaturateOnIntegerOverflow=on  OutDataTypeStr=Inherit: Same as input  ParamDataTypeStr=Inherit: Same as input
  rho : Constant  Value=1.205
  vMin : MinMax  Function=max  Inputs=2  InputSameDT=on  SaturateOnIntegerOverflow=on
  F_D : Outport  VectorParamsAs1DForOutWhenUnconnected=off
  PT.nEngine : Outport  Port=2  VectorParamsAs1DForOutWhenUnconnected=off
  wires:
  Sign/1 -> braking force/3
  Product2/1 -> PT.nEngine/1
  vMin/1 -> Product2/1
  Constant1/1 -> vMin/2
  Car.vx_1/1 -> Sign/1, Product4/1, Product4/2, vMin/1
  DM.Brake/1 -> mu/1
  "F_Mmax "/1 -> Product/2
  Look-Up Table/1 -> Product1/3
  Product1/1 -> Product/1, Product2/2
  Constant4/1 -> Product1/1
  Constant3/1 -> Product1/2
  Product/1 -> Sum/1
  DM.GearNo/1 -> Look-Up Table/1
  Sum/1 -> F_D/1
  braking force/1 -> Sum/2
  g/1 -> braking force/2
  m/1 -> g/1
  mu/1 -> braking force/1
  DM.Gas/1 -> "F_Mmax "/1
  A/1 -> Product3/5
  rho/1 -> Product3/4
  Constant6/1 -> Product3/3
  cW/1 -> Product3/2
  Product4/1 -> Product3/1
  Product3/1 -> Sum/3

== system SingleTrack/CarMaker/Vehicle/User Vehicle (CM4SL)/CarAndTrailer/single-track mass point model/yaw ==
  Steer.Ang : Inport
  Car.v : Inport  Port=2
  Car.v_dot : Inport  Port=3
  Car.mass : Inport  Port=4
  1/ J : Gain  Gain=1/1322.5  SaturateOnIntegerOverflow=on  OutDataTypeStr=Inherit: Same as input  ParamDataTypeStr=Inherit: Same as input
  Bus Selector : BusSelector  OutputSignals=Vhcl Cfg Yaw
  Multiply : Product  Inputs=**  OutDataTypeStr=double
  Sum : Sum  Inputs=+-  InputSameDT=on  SaturateOnIntegerOverflow=on  OutDataTypeStr=Inherit: Same as first input
  Sum1 : Sum  InputSameDT=on  SaturateOnIntegerOverflow=on  OutDataTypeStr=Inherit: Same as first input
  Vehicle Initial Cfg : Subsystem  mask(Vehicle Initial Configuration Values){}
      mask help: Provides some initial vehicle configuration values.
  aYaw * dt : Integrator  ExternalReset=level
  side forces : Subsystem
  sideslip angle : Subsystem
  vYaw * dt : Integrator  ExternalReset=level  InitialConditionSource=external
  beta : Outport  VectorParamsAs1DForOutWhenUnconnected=off
  beta_dot : Outport  Port=2  VectorParamsAs1DForOutWhenUnconnected=off
  Car.Yaw : Outport  Port=3  VectorParamsAs1DForOutWhenUnconnected=off
  Car.Yawp : Outport  Port=4  VectorParamsAs1DForOutWhenUnconnected=off
  Car.Yawpp : Outport  Port=5  VectorParamsAs1DForOutWhenUnconnected=off
  Car.Whl.F.SideSlip : Outport  Port=6  VectorParamsAs1DForOutWhenUnconnected=off
  Car.Whl.SideSlip : Outport  Port=7  VectorParamsAs1DForOutWhenUnconnected=off
  wires:
  Bus Selector/1 -> vYaw * dt/3  "<Vhcl Cfg Yaw>"
  side forces/6(alpha_R) -> Car.Whl.SideSlip/1
  side forces/5(alpha_F) -> Car.Whl.F.SideSlip/1
  sideslip angle/1(beta_dot) -> beta_dot/1
  Steer.Ang/1 -> side forces/4(StWhlAngle)
  sideslip angle/2(beta) -> beta/1, side forces/2(beta)
  Car.mass/1 -> sideslip angle/2(m)
  Car.v_dot/1 -> sideslip angle/3(v_dot)
  Sum1/1 -> sideslip angle/5(S)
  Sum/1 -> 1/ J/1
  side forces/1(S_F * l_F) -> Sum/1
  side forces/2(S_R * l_R) -> Sum/2
  1/ J/1 -> Car.Yawpp/1, aYaw * dt/1
  side forces/3(S_V) -> Sum1/1
  side forces/4(S_R) -> Sum1/2
  Car.v/1 -> sideslip angle/4(v), side forces/3(v)
  vYaw * dt/1 -> Car.Yaw/1
  Multiply/1 -> side forces/1(vYaw), sideslip angle/1(vYaw), vYaw * dt/1, Car.Yawp/1
  [TRStart] -> vYaw * dt/2, aYaw * dt/2
  aYaw * dt/1 -> Multiply/2
  [TRSim] -> Multiply/1
  Vehicle Initial Cfg/1(Vhcl.Cfg) -> Bus Selector/1

== system SingleTrack/CarMaker/Vehicle/User Vehicle (ModelMgr)/CarAndTrailer/CarAndTrailerUpd/CreateBus Brake.IF.In ==
  In : Inport
  BusCreator : BusCreator  Inputs=9
  Demux : Demux  Outputs=9
      settings: DisplayOption=none
  Out : Outport  VectorParamsAs1DForOutWhenUnconnected=off
  wires:
  Demux/9 -> BusCreator/9  "Brake IF Trq_Reg RR"
  Demux/8 -> BusCreator/8  "Brake IF Trq_Reg RL"
  Demux/7 -> BusCreator/7  "Brake IF Trq_Reg FR"
  Demux/6 -> BusCreator/6  "Brake IF Trq_Reg FL"
  Demux/5 -> BusCreator/5  "Brake IF Trq_Reg_max RR"
  Demux/4 -> BusCreator/4  "Brake IF Trq_Reg_max RL"
  Demux/3 -> BusCreator/3  "Brake IF Trq_Reg_max FR"
  Demux/2 -> BusCreator/2  "Brake IF Trq_Reg_max FL"
  Demux/1 -> BusCreator/1  "Brake IF T_env"
  BusCreator/1 -> Out/1
  In/1 -> Demux/1

== system SingleTrack/CarMaker/Vehicle/IPG Vehicle/CarAndTrailer/Forces/Suspension Forces/Buffer CreateBus CtrlOutOpt ==
  note: <Your model here>
  In : Inport
  Bus Creator{,1..3,9} (5 alike) : BusCreator  Inputs=4
  Demux{,2..5} (5 alike) : Demux
  Out : Outport
  wires:
  Bus Creator/1 -> Bus Creator9/1
  Demux/4 -> Demux5/1  "RR"
  Bus Creator2/1 -> Bus Creator9/3
  Demux5/1 -> Bus Creator3/1  "RR CtrlOutOpt0"
  Bus Creator3/1 -> Bus Creator9/4
  Demux2/4 -> Bus Creator/4  "FL CtrlOutOpt3"
  Demux5/3 -> Bus Creator3/3  "RR CtrlOutOpt2"
  Demux4/3 -> Bus Creator2/3  "RL CtrlOutOpt2"
  Bus Creator1/1 -> Bus Creator9/2
  Demux4/2 -> Bus Creator2/2  "RL CtrlOutOpt1"
  Demux2/2 -> Bus Creator/2  "FL CtrlOutOpt1"
  Demux/2 -> Demux3/1  "FR"
  Demux3/4 -> Bus Creator1/4  "FR CtrlOutOpt3"
  Demux3/1 -> Bus Creator1/1  "FR CtrlOutOpt0"
  Demux4/4 -> Bus Creator2/4  "RL CtrlOutOpt3"
  Demux2/3 -> Bus Creator/3  "FL CtrlOutOpt2"
  Demux3/2 -> Bus Creator1/2  "FR CtrlOutOpt1"
  Demux2/1 -> Bus Creator/1  "FL CtrlOutOpt0"
  Demux3/3 -> Bus Creator1/3  "FR CtrlOutOpt2"
  In/1 -> Demux/1
  Demux5/4 -> Bus Creator3/4  "RR CtrlOutOpt3"
  Demux/3 -> Demux4/1  "RL"
  Bus Creator9/1 -> Out/1
  Demux5/2 -> Bus Creator3/2  "RR CtrlOutOpt1"
  Demux4/1 -> Bus Creator2/1  "RL CtrlOutOpt0"
  Demux/1 -> Demux2/1  "FL"

== system SingleTrack/CarMaker/Vehicle/IPG Vehicle/CarAndTrailer/Forces/Suspension Forces/CreateBus BufferCtrlOutOpt ==
  note: <Your model here>
  In : Inport
  Bus Creator{,1..3,9} (5 alike) : BusCreator  Inputs=4
  Demux{,2..5} (5 alike) : Demux
  Out : Outport
  wires:
  Bus Creator/1 -> Bus Creator9/1
  Demux/4 -> Demux5/1  "RR"
  Bus Creator2/1 -> Bus Creator9/3
  Demux5/1 -> Bus Creator3/1  "RR CtrlOutOpt0"
  Bus Creator3/1 -> Bus Creator9/4
  Demux2/4 -> Bus Creator/4  "FL CtrlOutOpt3"
  Demux5/3 -> Bus Creator3/3  "RR CtrlOutOpt2"
  Demux4/3 -> Bus Creator2/3  "RL CtrlOutOpt2"
  Bus Creator1/1 -> Bus Creator9/2
  Demux4/2 -> Bus Creator2/2  "RL CtrlOutOpt1"
  Demux2/2 -> Bus Creator/2  "FL CtrlOutOpt1"
  Demux/2 -> Demux3/1  "FR"
  Demux3/4 -> Bus Creator1/4  "FR CtrlOutOpt3"
  Demux3/1 -> Bus Creator1/1  "FR CtrlOutOpt0"
  Demux4/4 -> Bus Creator2/4  "RL CtrlOutOpt3"
  Demux2/3 -> Bus Creator/3  "FL CtrlOutOpt2"
  Demux3/2 -> Bus Creator1/2  "FR CtrlOutOpt1"
  Demux2/1 -> Bus Creator/1  "FL CtrlOutOpt0"
  Demux3/3 -> Bus Creator1/3  "FR CtrlOutOpt2"
  Demux5/4 -> Bus Creator3/4  "RR CtrlOutOpt3"
  Demux/3 -> Demux4/1  "RL"
  Bus Creator9/1 -> Out/1
  Demux5/2 -> Bus Creator3/2  "RR CtrlOutOpt1"
  Demux4/1 -> Bus Creator2/1  "RL CtrlOutOpt0"
  Demux/1 -> Demux2/1  "FL"
  In/1 -> Demux/1

== system SingleTrack/CarMaker/Vehicle/IPG Vehicle/CarAndTrailer/Forces/Suspension Forces/CreateBus DamperCtrlOutOpt ==
  note: <Your model here>
  In : Inport
  Bus Creator{,1..3,9} (5 alike) : BusCreator  Inputs=4
  Demux{,2..5} (5 alike) : Demux
  Out : Outport
  wires:
  Bus Creator/1 -> Bus Creator9/1
  Demux/4 -> Demux5/1  "RR"
  Bus Creator2/1 -> Bus Creator9/3
  Demux5/1 -> Bus Creator3/1  "RR CtrlOutOpt0"
  Bus Creator3/1 -> Bus Creator9/4
  Demux2/4 -> Bus Creator/4  "FL CtrlOutOpt3"
  Demux5/3 -> Bus Creator3/3  "RR CtrlOutOpt2"
  Demux4/3 -> Bus Creator2/3  "RL CtrlOutOpt2"
  Bus Creator1/1 -> Bus Creator9/2
  Demux4/2 -> Bus Creator2/2  "RL CtrlOutOpt1"
  Demux2/2 -> Bus Creator/2  "FL CtrlOutOpt1"
  Demux/2 -> Demux3/1  "FR"
  Demux3/4 -> Bus Creator1/4  "FR CtrlOutOpt3"
  Demux3/1 -> Bus Creator1/1  "FR CtrlOutOpt0"
  Demux4/4 -> Bus Creator2/4  "RL CtrlOutOpt3"
  Demux2/3 -> Bus Creator/3  "FL CtrlOutOpt2"
  Demux3/2 -> Bus Creator1/2  "FR CtrlOutOpt1"
  Demux2/1 -> Bus Creator/1  "FL CtrlOutOpt0"
  Demux3/3 -> Bus Creator1/3  "FR CtrlOutOpt2"
  In/1 -> Demux/1
  Demux5/4 -> Bus Creator3/4  "RR CtrlOutOpt3"
  Demux/3 -> Demux4/1  "RL"
  Bus Creator9/1 -> Out/1
  Demux5/2 -> Bus Creator3/2  "RR CtrlOutOpt1"
  Demux4/1 -> Bus Creator2/1  "RL CtrlOutOpt0"
  Demux/1 -> Demux2/1  "FL"

== system SingleTrack/CarMaker/Vehicle/IPG Vehicle/CarAndTrailer/Forces/Suspension Forces/CreateBus FrcSystemCtrlOutOpt ==
  note: <Your model here>
  In : Inport
  Bus Creator9 : BusCreator  Inputs=64
  Demux : Demux  Outputs=64
  Out : Outport
  wires:
  In/1 -> Demux/1
  Bus Creator9/1 -> Out/1
  Demux/64 -> Bus Creator9/64  "CtrlOutOpt63"
  Demux/1 -> Bus Creator9/1  "CtrlOutOpt0"
  Demux/2 -> Bus Creator9/2  "CtrlOutOpt1"
  Demux/3 -> Bus Creator9/3  "CtrlOutOpt2"
  Demux/4 -> Bus Creator9/4  "CtrlOutOpt3"
  Demux/5 -> Bus Creator9/5  "CtrlOutOpt4"
  Demux/6 -> Bus Creator9/6  "CtrlOutOpt5"
  Demux/7 -> Bus Creator9/7  "CtrlOutOpt6"
  Demux/8 -> Bus Creator9/8  "CtrlOutOpt7"
  Demux/9 -> Bus Creator9/9  "CtrlOutOpt8"
  Demux/10 -> Bus Creator9/10  "CtrlOutOpt9"
  Demux/11 -> Bus Creator9/11  "CtrlOutOpt10"
  Demux/12 -> Bus Creator9/12  "CtrlOutOpt11"
  Demux/13 -> Bus Creator9/13  "CtrlOutOpt12"
  Demux/14 -> Bus Creator9/14  "CtrlOutOpt13"
  Demux/15 -> Bus Creator9/15  "CtrlOutOpt14"
  Demux/16 -> Bus Creator9/16  "CtrlOutOpt15"
  Demux/17 -> Bus Creator9/17  "CtrlOutOpt16"
  Demux/18 -> Bus Creator9/18  "CtrlOutOpt17"
  Demux/19 -> Bus Creator9/19  "CtrlOutOpt18"
  Demux/20 -> Bus Creator9/20  "CtrlOutOpt19"
  Demux/21 -> Bus Creator9/21  "CtrlOutOpt20"
  Demux/22 -> Bus Creator9/22  "CtrlOutOpt21"
  Demux/23 -> Bus Creator9/23  "CtrlOutOpt22"
  Demux/24 -> Bus Creator9/24  "CtrlOutOpt23"
  Demux/25 -> Bus Creator9/25  "CtrlOutOpt24"
  Demux/26 -> Bus Creator9/26  "CtrlOutOpt25"
  Demux/27 -> Bus Creator9/27  "CtrlOutOpt26"
  Demux/28 -> Bus Creator9/28  "CtrlOutOpt27"
  Demux/29 -> Bus Creator9/29  "CtrlOutOpt28"
  Demux/30 -> Bus Creator9/30  "CtrlOutOpt29"
  Demux/31 -> Bus Creator9/31  "CtrlOutOpt30"
  Demux/32 -> Bus Creator9/32  "CtrlOutOpt31"
  Demux/33 -> Bus Creator9/33  "CtrlOutOpt32"
  Demux/34 -> Bus Creator9/34  "CtrlOutOpt33"
  Demux/35 -> Bus Creator9/35  "CtrlOutOpt34"
  Demux/36 -> Bus Creator9/36  "CtrlOutOpt35"
  Demux/37 -> Bus Creator9/37  "CtrlOutOpt36"
  Demux/38 -> Bus Creator9/38  "CtrlOutOpt37"
  Demux/39 -> Bus Creator9/39  "CtrlOutOpt38"
  Demux/40 -> Bus Creator9/40  "CtrlOutOpt39"
  Demux/41 -> Bus Creator9/41  "CtrlOutOpt40"
  Demux/42 -> Bus Creator9/42  "CtrlOutOpt41"
  Demux/43 -> Bus Creator9/43  "CtrlOutOpt42"
  Demux/44 -> Bus Creator9/44  "CtrlOutOpt43"
  Demux/45 -> Bus Creator9/45  "CtrlOutOpt44"
  Demux/46 -> Bus Creator9/46  "CtrlOutOpt45"
  Demux/47 -> Bus Creator9/47  "CtrlOutOpt46"
  Demux/48 -> Bus Creator9/48  "CtrlOutOpt47"
  Demux/49 -> Bus Creator9/49  "CtrlOutOpt48"
  Demux/50 -> Bus Creator9/50  "CtrlOutOpt49"
  Demux/51 -> Bus Creator9/51  "CtrlOutOpt50"
  Demux/52 -> Bus Creator9/52  "CtrlOutOpt51"
  Demux/53 -> Bus Creator9/53  "CtrlOutOpt52"
  Demux/54 -> Bus Creator9/54  "CtrlOutOpt53"
  Demux/55 -> Bus Creator9/55  "CtrlOutOpt54"
  Demux/56 -> Bus Creator9/56  "CtrlOutOpt55"
  Demux/57 -> Bus Creator9/57  "CtrlOutOpt56"
  Demux/58 -> Bus Creator9/58  "CtrlOutOpt57"
  Demux/59 -> Bus Creator9/59  "CtrlOutOpt58"
  Demux/60 -> Bus Creator9/60  "CtrlOutOpt59"
  Demux/61 -> Bus Creator9/61  "CtrlOutOpt60"
  Demux/62 -> Bus Creator9/62  "CtrlOutOpt61"
  Demux/63 -> Bus Creator9/63  "CtrlOutOpt62"

== system SingleTrack/CarMaker/Vehicle/IPG Vehicle/CarAndTrailer/Forces/Suspension Forces/CreateBus SpringCtrlOutOpt ==
  note: <Your model here>
  In : Inport
  Bus Creator{,1..3,9} (5 alike) : BusCreator  Inputs=4
  Demux{,2..5} (5 alike) : Demux
  Out : Outport
  wires:
  Bus Creator/1 -> Bus Creator9/1
  Demux/4 -> Demux5/1  "RR"
  Bus Creator2/1 -> Bus Creator9/3
  Demux5/1 -> Bus Creator3/1  "RR CtrlOutOpt0"
  Bus Creator3/1 -> Bus Creator9/4
  Demux2/4 -> Bus Creator/4  "FL CtrlOutOpt3"
  Demux5/3 -> Bus Creator3/3  "RR CtrlOutOpt2"
  Demux4/3 -> Bus Creator2/3  "RL CtrlOutOpt2"
  Bus Creator1/1 -> Bus Creator9/2
  Demux4/2 -> Bus Creator2/2  "RL CtrlOutOpt1"
  Demux2/2 -> Bus Creator/2  "FL CtrlOutOpt1"
  Demux/2 -> Demux3/1  "FR"
  Demux3/4 -> Bus Creator1/4  "FR CtrlOutOpt3"
  Demux3/1 -> Bus Creator1/1  "FR CtrlOutOpt0"
  Demux4/4 -> Bus Creator2/4  "RL CtrlOutOpt3"
  Demux2/3 -> Bus Creator/3  "FL CtrlOutOpt2"
  Demux3/2 -> Bus Creator1/2  "FR CtrlOutOpt1"
  Demux2/1 -> Bus Creator/1  "FL CtrlOutOpt0"
  Demux3/3 -> Bus Creator1/3  "FR CtrlOutOpt2"
  In/1 -> Demux/1
  Demux5/4 -> Bus Creator3/4  "RR CtrlOutOpt3"
  Demux/3 -> Demux4/1  "RL"
  Bus Creator9/1 -> Out/1
  Demux5/2 -> Bus Creator3/2  "RR CtrlOutOpt1"
  Demux4/1 -> Bus Creator2/1  "RL CtrlOutOpt0"
  Demux/1 -> Demux2/1  "FL"
